simulink model "ALL_JP360_DBW_V6_5_1103"  (R2022a)
settings: Solver=FixedStepAuto  StartTime=0.0  StopTime=inf  FixedStep=0.01  RelTol=1e-3  EnableMultiTasking=on
model workspace (MAT data in the model file):
  g = 9.8
undefined symbols (not defined in the file or in its folder): canChannel, delta_v_p, IPM_Line_C0, IPM_Line_C1, IPM_Line_C2, IPM_Line_C3, M, M_p, MRR_ObjDistX, MRR_ObjDistY, MRR_ObjFusionCamID, MRR_ObjFusionSig, MRR_ObjID, MRR_ObjRelVelX, MRR_ObjRelVelY, MRR_ObjType, MRR_ObjUpdFlg, none, obj_vaild, untracktime, V, videoinput
libraries: canfdmsglib x230, canfdlib x76, slpidlib x24, simulink x18, dspstat3 x14, ctrlSharedLib x1, simulink_extras x1, imaqlib x1, realtime_pacer_lib x1, dspvision x1, visionsinks x1
(part 5 of 55)

== system ALL_JP360_DBW_V6_5_1103/MsgFromCAN/CCAN_GW_MsgFromCAN ==
  CCAN_GW_ABS_Sts_0x221FromInData : Inport  OutDataTypeStr=Bus:CAN_FD_MESSAGE_BUS
  CCAN_GW_ABS_Vspeed_0x601FromInData : Inport  Port=2  OutDataTypeStr=Bus:CAN_FD_MESSAGE_BUS
  CCAN_GW_ABS_WhlSpd_0x211FromInData : Inport  Port=3  OutDataTypeStr=Bus:CAN_FD_MESSAGE_BUS
  CCAN_GW_ADCU_0x538FromInData : Inport  Port=4  OutDataTypeStr=Bus:CAN_FD_MESSAGE_BUS
  CCAN_GW_ADCU_CanTSyn_0x570FromInData : Inport  Port=5  OutDataTypeStr=Bus:CAN_FD_MESSAGE_BUS
  CCAN_GW_BSD_0x275FromInData : Inport  Port=6  OutDataTypeStr=Bus:CAN_FD_MESSAGE_BUS
  CCAN_GW_EPS_0x260FromInData : Inport  Port=7  OutDataTypeStr=Bus:CAN_FD_MESSAGE_BUS
  CCAN_GW_EPS_Advanced_0x176FromInData : Inport  Port=8  OutDataTypeStr=Bus:CAN_FD_MESSAGE_BUS
  CCAN_GW_EPS_NM_0x5C2FromInData : Inport  Port=9  OutDataTypeStr=Bus:CAN_FD_MESSAGE_BUS
  CCAN_GW_ESP_Advanced_0x234FromInData : Inport  Port=10  OutDataTypeStr=Bus:CAN_FD_MESSAGE_BUS
  CCAN_GW_ESP_AxAy_0x242FromInData : Inport  Port=11  OutDataTypeStr=Bus:CAN_FD_MESSAGE_BUS
  CCAN_GW_ESP_Direction_0x235FromInData : Inport  Port=12  OutDataTypeStr=Bus:CAN_FD_MESSAGE_BUS
  CCAN_GW_ESP_OBD_Diag_0x600FromInData : Inport  Port=13  OutDataTypeStr=Bus:CAN_FD_MESSAGE_BUS
  CCAN_GW_ESP_Pressure_0x241FromInData : Inport  Port=14  OutDataTypeStr=Bus:CAN_FD_MESSAGE_BUS
  CCAN_GW_ESP_RAW_0x212FromInData : Inport  Port=15  OutDataTypeStr=Bus:CAN_FD_MESSAGE_BUS
  CCAN_GW_ESP_RPMF_0x213FromInData : Inport  Port=16  OutDataTypeStr=Bus:CAN_FD_MESSAGE_BUS
  CCAN_GW_ESP_RPMR_0x214FromInData : Inport  Port=17  OutDataTypeStr=Bus:CAN_FD_MESSAGE_BUS
  CCAN_GW_ESP_Status_0x243FromInData : Inport  Port=18  OutDataTypeStr=Bus:CAN_FD_MESSAGE_BUS
  CCAN_GW_ESP_Tq_0x217FromInData : Inport  Port=19  OutDataTypeStr=Bus:CAN_FD_MESSAGE_BUS
  CCAN_GW_GW_ESP_CCO_0x252FromInData : Inport  Port=20  OutDataTypeStr=Bus:CAN_FD_MESSAGE_BUS
  CCAN_GW_IPM_0x245FromInData : Inport  Port=21  OutDataTypeStr=Bus:CAN_FD_MESSAGE_BUS
  CCAN_GW_IPM_0x247FromInData : Inport  Port=22  OutDataTypeStr=Bus:CAN_FD_MESSAGE_BUS
  CCAN_GW_IPM_LeftLine_0x278FromInData : Inport  Port=23  OutDataTypeStr=Bus:CAN_FD_MESSAGE_BUS
  CCAN_GW_IPM_LeftLine_0x280FromInData : Inport  Port=24  OutDataTypeStr=Bus:CAN_FD_MESSAGE_BUS
  CCAN_GW_IPM_RightLine_0x490FromInData : Inport  Port=25  OutDataTypeStr=Bus:CAN_FD_MESSAGE_BUS
  CCAN_GW_IPM_RightLine_0x491FromInData : Inport  Port=26  OutDataTypeStr=Bus:CAN_FD_MESSAGE_BUS
  CCAN_GW_IPM_VLC_0x293FromInData : Inport  Port=27  OutDataTypeStr=Bus:CAN_FD_MESSAGE_BUS
  CCAN_GW_MRR_0x238FromInData : Inport  Port=28  OutDataTypeStr=Bus:CAN_FD_MESSAGE_BUS
  CCAN_GW_MRR_0x239FromInData : Inport  Port=29  OutDataTypeStr=Bus:CAN_FD_MESSAGE_BUS
  CCAN_GW_MRR_0x246FromInData : Inport  Port=30  OutDataTypeStr=Bus:CAN_FD_MESSAGE_BUS
  CCAN_GW_MRR_FRObj_0x279FromInData : Inport  Port=31  OutDataTypeStr=Bus:CAN_FD_MESSAGE_BUS
  CCAN_GW_MRR_LRObj_0x480FromInData : Inport  Port=32  OutDataTypeStr=Bus:CAN_FD_MESSAGE_BUS
  CCAN_GW_SAS_Sensor_0x175FromInData : Inport  Port=33  OutDataTypeStr=Bus:CAN_FD_MESSAGE_BUS
  CCAN_GW_SRR_FL_0x27BFromInData : Inport  Port=34  OutDataTypeStr=Bus:CAN_FD_MESSAGE_BUS
  CCAN_GW_SRR_RL_0x27AFromInData : Inport  Port=35  OutDataTypeStr=Bus:CAN_FD_MESSAGE_BUS
  CCAN_GW_ABS_Sts_0x221 : Subsystem  Commented=on  TreatAsAtomicUnit=on
  CCAN_GW_ABS_Vspeed_0x601 : Subsystem  Commented=on  TreatAsAtomicUnit=on
  CCAN_GW_ABS_WhlSpd_0x211 : Subsystem  Commented=on  TreatAsAtomicUnit=on
  CCAN_GW_ADCU_0x538 : Subsystem  Commented=on  TreatAsAtomicUnit=on
  CCAN_GW_ADCU_CanTSyn_0x570 : Subsystem  Commented=on  TreatAsAtomicUnit=on
  CCAN_GW_BSD_0x275 : Subsystem  Commented=on  TreatAsAtomicUnit=on
  CCAN_GW_EPS_0x260 : Subsystem  Commented=on  TreatAsAtomicUnit=on
  CCAN_GW_EPS_Advanced_0x176 : Subsystem  Commented=on  TreatAsAtomicUnit=on
  CCAN_GW_EPS_NM_0x5C2 : Subsystem  Commented=on  TreatAsAtomicUnit=on
  CCAN_GW_ESP_Advanced_0x234 : Subsystem  Commented=on  TreatAsAtomicUnit=on
  CCAN_GW_ESP_AxAy_0x242 : Subsystem  Commented=on  TreatAsAtomicUnit=on
  CCAN_GW_ESP_Direction_0x235 : Subsystem  Commented=on  TreatAsAtomicUnit=on
  CCAN_GW_ESP_OBD_Diag_0x600 : Subsystem  Commented=on  TreatAsAtomicUnit=on
  CCAN_GW_ESP_Pressure_0x241 : Subsystem  Commented=on  TreatAsAtomicUnit=on
  CCAN_GW_ESP_RAW_0x212 : Subsystem  Commented=on  TreatAsAtomicUnit=on
  CCAN_GW_ESP_RPMF_0x213 : Subsystem  Commented=on  TreatAsAtomicUnit=on
  CCAN_GW_ESP_RPMR_0x214 : Subsystem  Commented=on  TreatAsAtomicUnit=on
  CCAN_GW_ESP_Status_0x243 : Subsystem  Commented=on  TreatAsAtomicUnit=on
  CCAN_GW_ESP_Tq_0x217 : Subsystem  Commented=on  TreatAsAtomicUnit=on
  CCAN_GW_GW_ESP_CCO_0x252 : Subsystem  Commented=on  TreatAsAtomicUnit=on
  CCAN_GW_IPM_0x245 : Subsystem  Commented=on  TreatAsAtomicUnit=on
  CCAN_GW_IPM_0x247 : Subsystem  Commented=on  TreatAsAtomicUnit=on
  CCAN_GW_IPM_LeftLine_0x278 : Subsystem  Commented=on  TreatAsAtomicUnit=on
  CCAN_GW_IPM_LeftLine_0x280 : Subsystem  Commented=on  TreatAsAtomicUnit=on
  CCAN_GW_IPM_RightLine_0x490 : Subsystem  Commented=on  TreatAsAtomicUnit=on
  CCAN_GW_IPM_RightLine_0x491 : Subsystem  Commented=on  TreatAsAtomicUnit=on
  CCAN_GW_IPM_VLC_0x293 : Subsystem  Commented=on  TreatAsAtomicUnit=on
  CCAN_GW_MRR_0x238 : Subsystem  Commented=on  TreatAsAtomicUnit=on
  CCAN_GW_MRR_0x239 : Subsystem  Commented=on  TreatAsAtomicUnit=on
  CCAN_GW_MRR_0x246 : Subsystem  TreatAsAtomicUnit=on
  CCAN_GW_MRR_FRObj_0x279 : Subsystem  TreatAsAtomicUnit=on
  CCAN_GW_MRR_LRObj_0x480 : Subsystem  Commented=on  TreatAsAtomicUnit=on
  CCAN_GW_SAS_Sensor_0x175 : Subsystem  Commented=on  TreatAsAtomicUnit=on
  CCAN_GW_SRR_FL_0x27B : Subsystem  Commented=on  TreatAsAtomicUnit=on
  CCAN_GW_SRR_RL_0x27A : Subsystem  Commented=on  TreatAsAtomicUnit=on
  CCAN_GW_ABS_Sts_0x221FromOutData : Outport  OutDataTypeStr=Bus:CCAN_GW_ABS_Sts_0x221
  CCAN_GW_ABS_Vspeed_0x601FromOutData : Outport  Port=2  OutDataTypeStr=Bus:CCAN_GW_ABS_Vspeed_0x601
  CCAN_GW_ABS_WhlSpd_0x211FromOutData : Outport  Port=3  OutDataTypeStr=Bus:CCAN_GW_ABS_WhlSpd_0x211
  CCAN_GW_ADCU_0x538FromOutData : Outport  Port=4  OutDataTypeStr=Bus:CCAN_GW_ADCU_0x538
  CCAN_GW_ADCU_CanTSyn_0x570FromOutData : Outport  Port=5  OutDataTypeStr=Bus:CCAN_GW_ADCU_CanTSyn_0x570
  CCAN_GW_BSD_0x275FromOutData : Outport  Port=6  OutDataTypeStr=Bus:CCAN_GW_BSD_0x275
  CCAN_GW_EPS_0x260FromOutData : Outport  Port=7  OutDataTypeStr=Bus:CCAN_GW_EPS_0x260
  CCAN_GW_EPS_Advanced_0x176FromOutData : Outport  Port=8  OutDataTypeStr=Bus:CCAN_GW_EPS_Advanced_0x176
  CCAN_GW_EPS_NM_0x5C2FromOutData : Outport  Port=9  OutDataTypeStr=Bus:CCAN_GW_EPS_NM_0x5C2
  CCAN_GW_ESP_Advanced_0x234FromOutData : Outport  Port=10  OutDataTypeStr=Bus:CCAN_GW_ESP_Advanced_0x234
  CCAN_GW_ESP_AxAy_0x242FromOutData : Outport  Port=11  OutDataTypeStr=Bus:CCAN_GW_ESP_AxAy_0x242
  CCAN_GW_ESP_Direction_0x235FromOutData : Outport  Port=12  OutDataTypeStr=Bus:CCAN_GW_ESP_Direction_0x235
  CCAN_GW_ESP_OBD_Diag_0x600FromOutData : Outport  Port=13  OutDataTypeStr=Bus:CCAN_GW_ESP_OBD_Diag_0x600
  CCAN_GW_ESP_Pressure_0x241FromOutData : Outport  Port=14  OutDataTypeStr=Bus:CCAN_GW_ESP_Pressure_0x241
  CCAN_GW_ESP_RAW_0x212FromOutData : Outport  Port=15  OutDataTypeStr=Bus:CCAN_GW_ESP_RAW_0x212
  CCAN_GW_ESP_RPMF_0x213FromOutData : Outport  Port=16  OutDataTypeStr=Bus:CCAN_GW_ESP_RPMF_0x213
  CCAN_GW_ESP_RPMR_0x214FromOutData : Outport  Port=17  OutDataTypeStr=Bus:CCAN_GW_ESP_RPMR_0x214
  CCAN_GW_ESP_Status_0x243FromOutData : Outport  Port=18  OutDataTypeStr=Bus:CCAN_GW_ESP_Status_0x243
  CCAN_GW_ESP_Tq_0x217FromOutData : Outport  Port=19  OutDataTypeStr=Bus:CCAN_GW_ESP_Tq_0x217
  CCAN_GW_GW_ESP_CCO_0x252FromOutData : Outport  Port=20  OutDataTypeStr=Bus:CCAN_GW_GW_ESP_CCO_0x252
  CCAN_GW_IPM_0x245FromOutData : Outport  Port=21  OutDataTypeStr=Bus:CCAN_GW_IPM_0x245
  CCAN_GW_IPM_0x247FromOutData : Outport  Port=22  OutDataTypeStr=Bus:CCAN_GW_IPM_0x247
  CCAN_GW_IPM_LeftLine_0x278FromOutData : Outport  Port=23  OutDataTypeStr=Bus:CCAN_GW_IPM_LeftLine_0x278
  CCAN_GW_IPM_LeftLine_0x280FromOutData : Outport  Port=24  OutDataTypeStr=Bus:CCAN_GW_IPM_LeftLine_0x280
  CCAN_GW_IPM_RightLine_0x490FromOutData : Outport  Port=25  OutDataTypeStr=Bus:CCAN_GW_IPM_RightLine_0x490
  CCAN_GW_IPM_RightLine_0x491FromOutData : Outport  Port=26  OutDataTypeStr=Bus:CCAN_GW_IPM_RightLine_0x491
  CCAN_GW_IPM_VLC_0x293FromOutData : Outport  Port=27  OutDataTypeStr=Bus:CCAN_GW_IPM_VLC_0x293
  CCAN_GW_MRR_0x238FromOutData : Outport  Port=28  OutDataTypeStr=Bus:CCAN_GW_MRR_0x238
  CCAN_GW_MRR_0x239FromOutData : Outport  Port=29  OutDataTypeStr=Bus:CCAN_GW_MRR_0x239
  CCAN_GW_MRR_0x246FromOutData : Outport  Port=30  OutDataTypeStr=Bus:CCAN_GW_MRR_0x246
  CCAN_GW_MRR_FRObj_0x279FromOutData : Outport  Port=31  OutDataTypeStr=Bus:CCAN_GW_MRR_FRObj_0x279
  CCAN_GW_MRR_LRObj_0x480FromOutData : Outport  Port=32  OutDataTypeStr=Bus:CCAN_GW_MRR_LRObj_0x480
  CCAN_GW_SAS_Sensor_0x175FromOutData : Outport  Port=33  OutDataTypeStr=Bus:CCAN_GW_SAS_Sensor_0x175
  CCAN_GW_SRR_FL_0x27BFromOutData : Outport  Port=34  OutDataTypeStr=Bus:CCAN_GW_SRR_FL_0x27B
  CCAN_GW_SRR_RL_0x27AFromOutData : Outport  Port=35  OutDataTypeStr=Bus:CCAN_GW_SRR_RL_0x27A
  wires:
  CCAN_GW_ABS_Sts_0x221/1(CCAN_GW_ABS_Sts_0x221FromOutData) -> CCAN_GW_ABS_Sts_0x221FromOutData/1  "CCAN_GW_ABS_Sts_0x221FromOutData"
  CCAN_GW_ABS_Sts_0x221FromInData/1 -> CCAN_GW_ABS_Sts_0x221/1(CCAN_GW_ABS_Sts_0x221FromInData)  "CCAN_GW_ABS_Sts_0x221FromInData"
  CCAN_GW_ABS_Vspeed_0x601/1(CCAN_GW_ABS_Vspeed_0x601FromOutData) -> CCAN_GW_ABS_Vspeed_0x601FromOutData/1  "CCAN_GW_ABS_Vspeed_0x601FromOutData"
  CCAN_GW_ABS_Vspeed_0x601FromInData/1 -> CCAN_GW_ABS_Vspeed_0x601/1(CCAN_GW_ABS_Vspeed_0x601FromInData)  "CCAN_GW_ABS_Vspeed_0x601FromInData"
  CCAN_GW_ABS_WhlSpd_0x211/1(CCAN_GW_ABS_WhlSpd_0x211FromOutData) -> CCAN_GW_ABS_WhlSpd_0x211FromOutData/1  "CCAN_GW_ABS_WhlSpd_0x211FromOutData"
  CCAN_GW_ABS_WhlSpd_0x211FromInData/1 -> CCAN_GW_ABS_WhlSpd_0x211/1(CCAN_GW_ABS_WhlSpd_0x211FromInData)  "CCAN_GW_ABS_WhlSpd_0x211FromInData"
  CCAN_GW_ADCU_0x538/1(CCAN_GW_ADCU_0x538FromOutData) -> CCAN_GW_ADCU_0x538FromOutData/1  "CCAN_GW_ADCU_0x538FromOutData"
  CCAN_GW_ADCU_0x538FromInData/1 -> CCAN_GW_ADCU_0x538/1(CCAN_GW_ADCU_0x538FromInData)  "CCAN_GW_ADCU_0x538FromInData"
  CCAN_GW_ADCU_CanTSyn_0x570/1(CCAN_GW_ADCU_CanTSyn_0x570FromOutData) -> CCAN_GW_ADCU_CanTSyn_0x570FromOutData/1  "CCAN_GW_ADCU_CanTSyn_0x570FromOutData"
  CCAN_GW_ADCU_CanTSyn_0x570FromInData/1 -> CCAN_GW_ADCU_CanTSyn_0x570/1(CCAN_GW_ADCU_CanTSyn_0x570FromInData)  "CCAN_GW_ADCU_CanTSyn_0x570FromInData"
  CCAN_GW_BSD_0x275/1(CCAN_GW_BSD_0x275FromOutData) -> CCAN_GW_BSD_0x275FromOutData/1  "CCAN_GW_BSD_0x275FromOutData"
  CCAN_GW_BSD_0x275FromInData/1 -> CCAN_GW_BSD_0x275/1(CCAN_GW_BSD_0x275FromInData)  "CCAN_GW_BSD_0x275FromInData"
  CCAN_GW_EPS_0x260/1(CCAN_GW_EPS_0x260FromOutData) -> CCAN_GW_EPS_0x260FromOutData/1  "CCAN_GW_EPS_0x260FromOutData"
  CCAN_GW_EPS_0x260FromInData/1 -> CCAN_GW_EPS_0x260/1(CCAN_GW_EPS_0x260FromInData)  "CCAN_GW_EPS_0x260FromInData"
  CCAN_GW_EPS_Advanced_0x176/1(CCAN_GW_EPS_Advanced_0x176FromOutData) -> CCAN_GW_EPS_Advanced_0x176FromOutData/1  "CCAN_GW_EPS_Advanced_0x176FromOutData"
  CCAN_GW_EPS_Advanced_0x176FromInData/1 -> CCAN_GW_EPS_Advanced_0x176/1(CCAN_GW_EPS_Advanced_0x176FromInData)  "CCAN_GW_EPS_Advanced_0x176FromInData"
  CCAN_GW_EPS_NM_0x5C2/1(CCAN_GW_EPS_NM_0x5C2FromOutData) -> CCAN_GW_EPS_NM_0x5C2FromOutData/1  "CCAN_GW_EPS_NM_0x5C2FromOutData"
  CCAN_GW_EPS_NM_0x5C2FromInData/1 -> CCAN_GW_EPS_NM_0x5C2/1(CCAN_GW_EPS_NM_0x5C2FromInData)  "CCAN_GW_EPS_NM_0x5C2FromInData"
  CCAN_GW_ESP_Advanced_0x234/1(CCAN_GW_ESP_Advanced_0x234FromOutData) -> CCAN_GW_ESP_Advanced_0x234FromOutData/1  "CCAN_GW_ESP_Advanced_0x234FromOutData"
  CCAN_GW_ESP_Advanced_0x234FromInData/1 -> CCAN_GW_ESP_Advanced_0x234/1(CCAN_GW_ESP_Advanced_0x234FromInData)  "CCAN_GW_ESP_Advanced_0x234FromInData"
  CCAN_GW_ESP_AxAy_0x242/1(CCAN_GW_ESP_AxAy_0x242FromOutData) -> CCAN_GW_ESP_AxAy_0x242FromOutData/1  "CCAN_GW_ESP_AxAy_0x242FromOutData"
  CCAN_GW_ESP_AxAy_0x242FromInData/1 -> CCAN_GW_ESP_AxAy_0x242/1(CCAN_GW_ESP_AxAy_0x242FromInData)  "CCAN_GW_ESP_AxAy_0x242FromInData"
  CCAN_GW_ESP_Direction_0x235/1(CCAN_GW_ESP_Direction_0x235FromOutData) -> CCAN_GW_ESP_Direction_0x235FromOutData/1  "CCAN_GW_ESP_Direction_0x235FromOutData"
  CCAN_GW_ESP_Direction_0x235FromInData/1 -> CCAN_GW_ESP_Direction_0x235/1(CCAN_GW_ESP_Direction_0x235FromInData)  "CCAN_GW_ESP_Direction_0x235FromInData"
  CCAN_GW_ESP_OBD_Diag_0x600/1(CCAN_GW_ESP_OBD_Diag_0x600FromOutData) -> CCAN_GW_ESP_OBD_Diag_0x600FromOutData/1  "CCAN_GW_ESP_OBD_Diag_0x600FromOutData"
  CCAN_GW_ESP_OBD_Diag_0x600FromInData/1 -> CCAN_GW_ESP_OBD_Diag_0x600/1(CCAN_GW_ESP_OBD_Diag_0x600FromInData)  "CCAN_GW_ESP_OBD_Diag_0x600FromInData"
  CCAN_GW_ESP_Pressure_0x241/1(CCAN_GW_ESP_Pressure_0x241FromOutData) -> CCAN_GW_ESP_Pressure_0x241FromOutData/1  "CCAN_GW_ESP_Pressure_0x241FromOutData"
  CCAN_GW_ESP_Pressure_0x241FromInData/1 -> CCAN_GW_ESP_Pressure_0x241/1(CCAN_GW_ESP_Pressure_0x241FromInData)  "CCAN_GW_ESP_Pressure_0x241FromInData"
  CCAN_GW_ESP_RAW_0x212/1(CCAN_GW_ESP_RAW_0x212FromOutData) -> CCAN_GW_ESP_RAW_0x212FromOutData/1  "CCAN_GW_ESP_RAW_0x212FromOutData"
  CCAN_GW_ESP_RAW_0x212FromInData/1 -> CCAN_GW_ESP_RAW_0x212/1(CCAN_GW_ESP_RAW_0x212FromInData)  "CCAN_GW_ESP_RAW_0x212FromInData"
  CCAN_GW_ESP_RPMF_0x213/1(CCAN_GW_ESP_RPMF_0x213FromOutData) -> CCAN_GW_ESP_RPMF_0x213FromOutData/1  "CCAN_GW_ESP_RPMF_0x213FromOutData"
  CCAN_GW_ESP_RPMF_0x213FromInData/1 -> CCAN_GW_ESP_RPMF_0x213/1(CCAN_GW_ESP_RPMF_0x213FromInData)  "CCAN_GW_ESP_RPMF_0x213FromInData"
  CCAN_GW_ESP_RPMR_0x214/1(CCAN_GW_ESP_RPMR_0x214FromOutData) -> CCAN_GW_ESP_RPMR_0x214FromOutData/1  "CCAN_GW_ESP_RPMR_0x214FromOutData"
  CCAN_GW_ESP_RPMR_0x214FromInData/1 -> CCAN_GW_ESP_RPMR_0x214/1(CCAN_GW_ESP_RPMR_0x214FromInData)  "CCAN_GW_ESP_RPMR_0x214FromInData"
  CCAN_GW_ESP_Status_0x243/1(CCAN_GW_ESP_Status_0x243FromOutData) -> CCAN_GW_ESP_Status_0x243FromOutData/1  "CCAN_GW_ESP_Status_0x243FromOutData"
  CCAN_GW_ESP_Status_0x243FromInData/1 -> CCAN_GW_ESP_Status_0x243/1(CCAN_GW_ESP_Status_0x243FromInData)  "CCAN_GW_ESP_Status_0x243FromInData"
  CCAN_GW_ESP_Tq_0x217/1(CCAN_GW_ESP_Tq_0x217FromOutData) -> CCAN_GW_ESP_Tq_0x217FromOutData/1  "CCAN_GW_ESP_Tq_0x217FromOutData"
  CCAN_GW_ESP_Tq_0x217FromInData/1 -> CCAN_GW_ESP_Tq_0x217/1(CCAN_GW_ESP_Tq_0x217FromInData)  "CCAN_GW_ESP_Tq_0x217FromInData"
  CCAN_GW_GW_ESP_CCO_0x252/1(CCAN_GW_GW_ESP_CCO_0x252FromOutData) -> CCAN_GW_GW_ESP_CCO_0x252FromOutData/1  "CCAN_GW_GW_ESP_CCO_0x252FromOutData"
  CCAN_GW_GW_ESP_CCO_0x252FromInData/1 -> CCAN_GW_GW_ESP_CCO_0x252/1(CCAN_GW_GW_ESP_CCO_0x252FromInData)  "CCAN_GW_GW_ESP_CCO_0x252FromInData"
  CCAN_GW_IPM_0x245/1(CCAN_GW_IPM_0x245FromOutData) -> CCAN_GW_IPM_0x245FromOutData/1  "CCAN_GW_IPM_0x245FromOutData"
  CCAN_GW_IPM_0x245FromInData/1 -> CCAN_GW_IPM_0x245/1(CCAN_GW_IPM_0x245FromInData)  "CCAN_GW_IPM_0x245FromInData"
  CCAN_GW_IPM_0x247/1(CCAN_GW_IPM_0x247FromOutData) -> CCAN_GW_IPM_0x247FromOutData/1  "CCAN_GW_IPM_0x247FromOutData"
  CCAN_GW_IPM_0x247FromInData/1 -> CCAN_GW_IPM_0x247/1(CCAN_GW_IPM_0x247FromInData)  "CCAN_GW_IPM_0x247FromInData"
  CCAN_GW_IPM_LeftLine_0x278/1(CCAN_GW_IPM_LeftLine_0x278FromOutData) -> CCAN_GW_IPM_LeftLine_0x278FromOutData/1  "CCAN_GW_IPM_LeftLine_0x278FromOutData"
  CCAN_GW_IPM_LeftLine_0x278FromInData/1 -> CCAN_GW_IPM_LeftLine_0x278/1(CCAN_GW_IPM_LeftLine_0x278FromInData)  "CCAN_GW_IPM_LeftLine_0x278FromInData"
  CCAN_GW_IPM_LeftLine_0x280/1(CCAN_GW_IPM_LeftLine_0x280FromOutData) -> CCAN_GW_IPM_LeftLine_0x280FromOutData/1  "CCAN_GW_IPM_LeftLine_0x280FromOutData"
  CCAN_GW_IPM_LeftLine_0x280FromInData/1 -> CCAN_GW_IPM_LeftLine_0x280/1(CCAN_GW_IPM_LeftLine_0x280FromInData)  "CCAN_GW_IPM_LeftLine_0x280FromInData"
  CCAN_GW_IPM_RightLine_0x490/1(CCAN_GW_IPM_RightLine_0x490FromOutData) -> CCAN_GW_IPM_RightLine_0x490FromOutData/1  "CCAN_GW_IPM_RightLine_0x490FromOutData"
  CCAN_GW_IPM_RightLine_0x490FromInData/1 -> CCAN_GW_IPM_RightLine_0x490/1(CCAN_GW_IPM_RightLine_0x490FromInData)  "CCAN_GW_IPM_RightLine_0x490FromInData"
  CCAN_GW_IPM_RightLine_0x491/1(CCAN_GW_IPM_RightLine_0x491FromOutData) -> CCAN_GW_IPM_RightLine_0x491FromOutData/1  "CCAN_GW_IPM_RightLine_0x491FromOutData"
  CCAN_GW_IPM_RightLine_0x491FromInData/1 -> CCAN_GW_IPM_RightLine_0x491/1(CCAN_GW_IPM_RightLine_0x491FromInData)  "CCAN_GW_IPM_RightLine_0x491FromInData"
  CCAN_GW_IPM_VLC_0x293/1(CCAN_GW_IPM_VLC_0x293FromOutData) -> CCAN_GW_IPM_VLC_0x293FromOutData/1  "CCAN_GW_IPM_VLC_0x293FromOutData"
  CCAN_GW_IPM_VLC_0x293FromInData/1 -> CCAN_GW_IPM_VLC_0x293/1(CCAN_GW_IPM_VLC_0x293FromInData)  "CCAN_GW_IPM_VLC_0x293FromInData"
  CCAN_GW_MRR_0x238/1(CCAN_GW_MRR_0x238FromOutData) -> CCAN_GW_MRR_0x238FromOutData/1  "CCAN_GW_MRR_0x238FromOutData"
  CCAN_GW_MRR_0x238FromInData/1 -> CCAN_GW_MRR_0x238/1(CCAN_GW_MRR_0x238FromInData)  "CCAN_GW_MRR_0x238FromInData"
  CCAN_GW_MRR_0x239/1(CCAN_GW_MRR_0x239FromOutData) -> CCAN_GW_MRR_0x239FromOutData/1  "CCAN_GW_MRR_0x239FromOutData"
  CCAN_GW_MRR_0x239FromInData/1 -> CCAN_GW_MRR_0x239/1(CCAN_GW_MRR_0x239FromInData)  "CCAN_GW_MRR_0x239FromInData"
  CCAN_GW_MRR_0x246/1(CCAN_GW_MRR_0x246FromOutData) -> CCAN_GW_MRR_0x246FromOutData/1  "CCAN_GW_MRR_0x246FromOutData"
  CCAN_GW_MRR_0x246FromInData/1 -> CCAN_GW_MRR_0x246/1(CCAN_GW_MRR_0x246FromInData)  "CCAN_GW_MRR_0x246FromInData"
  CCAN_GW_MRR_FRObj_0x279/1(CCAN_GW_MRR_FRObj_0x279FromOutData) -> CCAN_GW_MRR_FRObj_0x279FromOutData/1  "CCAN_GW_MRR_FRObj_0x279FromOutData"
  CCAN_GW_MRR_FRObj_0x279FromInData/1 -> CCAN_GW_MRR_FRObj_0x279/1(CCAN_GW_MRR_FRObj_0x279FromInData)  "CCAN_GW_MRR_FRObj_0x279FromInData"
  CCAN_GW_MRR_LRObj_0x480/1(CCAN_GW_MRR_LRObj_0x480FromOutData) -> CCAN_GW_MRR_LRObj_0x480FromOutData/1  "CCAN_GW_MRR_LRObj_0x480FromOutData"
  CCAN_GW_MRR_LRObj_0x480FromInData/1 -> CCAN_GW_MRR_LRObj_0x480/1(CCAN_GW_MRR_LRObj_0x480FromInData)  "CCAN_GW_MRR_LRObj_0x480FromInData"
  CCAN_GW_SAS_Sensor_0x175/1(CCAN_GW_SAS_Sensor_0x175FromOutData) -> CCAN_GW_SAS_Sensor_0x175FromOutData/1  "CCAN_GW_SAS_Sensor_0x175FromOutData"
  CCAN_GW_SAS_Sensor_0x175FromInData/1 -> CCAN_GW_SAS_Sensor_0x175/1(CCAN_GW_SAS_Sensor_0x175FromInData)  "CCAN_GW_SAS_Sensor_0x175FromInData"
  CCAN_GW_SRR_FL_0x27B/1(CCAN_GW_SRR_FL_0x27BFromOutData) -> CCAN_GW_SRR_FL_0x27BFromOutData/1  "CCAN_GW_SRR_FL_0x27BFromOutData"
  CCAN_GW_SRR_FL_0x27BFromInData/1 -> CCAN_GW_SRR_FL_0x27B/1(CCAN_GW_SRR_FL_0x27BFromInData)  "CCAN_GW_SRR_FL_0x27BFromInData"
  CCAN_GW_SRR_RL_0x27A/1(CCAN_GW_SRR_RL_0x27AFromOutData) -> CCAN_GW_SRR_RL_0x27AFromOutData/1  "CCAN_GW_SRR_RL_0x27AFromOutData"
  CCAN_GW_SRR_RL_0x27AFromInData/1 -> CCAN_GW_SRR_RL_0x27A/1(CCAN_GW_SRR_RL_0x27AFromInData)  "CCAN_GW_SRR_RL_0x27AFromInData"

== system ALL_JP360_DBW_V6_5_1103/MsgFromCAN/IPM_Line_data ==
  CAN FD Receive1 : canfdlib/CAN FD Receive  BlockHandle=84597.0006  Device=Vector VN1640A 1 (Channel 4)  ObjConstructor=canChannel('Vector', 'VN1640A 1', 4, 'ProtocolMode', 'CAN FD')  EnableStandardIDsFilter=off  StdIDsCombo=Allow only  StandardIDs=1600  EnableExtendedIDsFilter=off  ExtIDsCombo=Allow all  ExtendedIDs=0  SampleTime=0.01  MsgsPerTimestep=all  InternalFilterUpdateStatus=on  BusOutput=on
      settings: SourceProductBaseCode=VN
  CAN FD Receive2 : canfdlib/CAN FD Receive  BlockHandle=84600.0006  Device=Vector VN1640A 1 (Channel 4)  ObjConstructor=canChannel('Vector', 'VN1640A 1', 4, 'ProtocolMode', 'CAN FD')  EnableStandardIDsFilter=off  StdIDsCombo=Allow only  StandardIDs=1601  EnableExtendedIDsFilter=off  ExtIDsCombo=Allow all  ExtendedIDs=0  SampleTime=0.01  MsgsPerTimestep=all  InternalFilterUpdateStatus=on  BusOutput=on
      settings: SourceProductBaseCode=VN
  CAN FD Receive3 : canfdlib/CAN FD Receive  BlockHandle=84603.0006  Device=Vector VN1640A 1 (Channel 4)  ObjConstructor=canChannel('Vector', 'VN1640A 1', 4, 'ProtocolMode', 'CAN FD')  EnableStandardIDsFilter=off  StdIDsCombo=Allow only  StandardIDs=1602  EnableExtendedIDsFilter=off  ExtIDsCombo=Allow all  ExtendedIDs=0  SampleTime=0.01  MsgsPerTimestep=all  InternalFilterUpdateStatus=on  BusOutput=on
      settings: SourceProductBaseCode=VN
  CAN FD Receive4 : canfdlib/CAN FD Receive  BlockHandle=84606.0006  Device=Vector VN1640A 1 (Channel 4)  ObjConstructor=canChannel('Vector', 'VN1640A 1', 4, 'ProtocolMode', 'CAN FD')  EnableStandardIDsFilter=off  StdIDsCombo=Allow only  StandardIDs=1603  EnableExtendedIDsFilter=off  ExtIDsCombo=Allow all  ExtendedIDs=0  SampleTime=0.01  MsgsPerTimestep=all  InternalFilterUpdateStatus=on  BusOutput=on
      settings: SourceProductBaseCode=VN
  Terminator{16..19} (4 alike) : Terminator
  VR_ADCU_IPM_Line_01_0x640FromInData : Outport
  VR_ADCU_IPM_Line_02_0x641FromInData : Outport  Port=2
  VR_ADCU_IPM_Line_03_0x642FromInData : Outport  Port=3
  VR_ADCU_IPM_Line_04_0x643FromInData : Outport  Port=4
  wires:
  CAN FD Receive4/1 -> Terminator19/1
  CAN FD Receive3/1 -> Terminator18/1
  CAN FD Receive3/2 -> VR_ADCU_IPM_Line_03_0x642FromInData/1
  CAN FD Receive1/1 -> Terminator16/1
  CAN FD Receive4/2 -> VR_ADCU_IPM_Line_04_0x643FromInData/1
  CAN FD Receive2/1 -> Terminator17/1
  CAN FD Receive2/2 -> VR_ADCU_IPM_Line_02_0x641FromInData/1
  CAN FD Receive1/2 -> VR_ADCU_IPM_Line_01_0x640FromInData/1

== system ALL_JP360_DBW_V6_5_1103/MsgFromCAN/IPM_Obj_data ==
  CAN FD Receive1 : canfdlib/CAN FD Receive  BlockHandle=84647.0004  Device=Vector VN1640A 1 (Channel 4)  ObjConstructor=canChannel('Vector', 'VN1640A 1', 4, 'ProtocolMode', 'CAN FD')  EnableStandardIDsFilter=off  StdIDsCombo=Allow only  StandardIDs=1616  EnableExtendedIDsFilter=off  ExtIDsCombo=Allow all  ExtendedIDs=0  SampleTime=0.01  MsgsPerTimestep=all  InternalFilterUpdateStatus=on  BusOutput=on
      settings: SourceProductBaseCode=VN
  CAN FD Receive10 : canfdlib/CAN FD Receive  BlockHandle=84650.0004  Device=Vector VN1640A 1 (Channel 4)  ObjConstructor=canChannel('Vector', 'VN1640A 1', 4, 'ProtocolMode', 'CAN FD')  EnableStandardIDsFilter=off  StdIDsCombo=Allow only  StandardIDs=1625  EnableExtendedIDsFilter=off  ExtIDsCombo=Allow all  ExtendedIDs=0  SampleTime=0.01  MsgsPerTimestep=all  InternalFilterUpdateStatus=on  BusOutput=on
      settings: SourceProductBaseCode=VN
  CAN FD Receive11 : canfdlib/CAN FD Receive  BlockHandle=84653.0004  Device=Vector VN1640A 1 (Channel 4)  ObjConstructor=canChannel('Vector', 'VN1640A 1', 4, 'ProtocolMode', 'CAN FD')  EnableStandardIDsFilter=off  StdIDsCombo=Allow only  StandardIDs=1626  EnableExtendedIDsFilter=off  ExtIDsCombo=Allow all  ExtendedIDs=0  SampleTime=0.01  MsgsPerTimestep=all  InternalFilterUpdateStatus=on  BusOutput=on
      settings: SourceProductBaseCode=VN
  CAN FD Receive12 : canfdlib/CAN FD Receive  BlockHandle=84656.0005  Device=Vector VN1640A 1 (Channel 4)  ObjConstructor=canChannel('Vector', 'VN1640A 1', 4, 'ProtocolMode', 'CAN FD')  EnableStandardIDsFilter=off  StdIDsCombo=Allow only  StandardIDs=1627  EnableExtendedIDsFilter=off  ExtIDsCombo=Allow all  ExtendedIDs=0  SampleTime=0.01  MsgsPerTimestep=all  InternalFilterUpdateStatus=on  BusOutput=on
      settings: SourceProductBaseCode=VN
  CAN FD Receive13 : canfdlib/CAN FD Receive  BlockHandle=84659.0012  Device=Vector VN1640A 1 (Channel 4)  ObjConstructor=canChannel('Vector', 'VN1640A 1', 4, 'ProtocolMode', 'CAN FD')  EnableStandardIDsFilter=off  StdIDsCombo=Allow only  StandardIDs=1628  EnableExtendedIDsFilter=off  ExtIDsCombo=Allow all  ExtendedIDs=0  SampleTime=0.01  MsgsPerTimestep=all  InternalFilterUpdateStatus=on  BusOutput=on
      settings: SourceProductBaseCode=VN
  CAN FD Receive14 : canfdlib/CAN FD Receive  BlockHandle=84662.0005  Device=Vector VN1640A 1 (Channel 4)  ObjConstructor=canChannel('Vector', 'VN1640A 1', 4, 'ProtocolMode', 'CAN FD')  EnableStandardIDsFilter=off  StdIDsCombo=Allow only  StandardIDs=1629  EnableExtendedIDsFilter=off  ExtIDsCombo=Allow all  ExtendedIDs=0  SampleTime=0.01  MsgsPerTimestep=all  InternalFilterUpdateStatus=on  BusOutput=on
      settings: SourceProductBaseCode=VN
  CAN FD Receive15 : canfdlib/CAN FD Receive  BlockHandle=84665.0004  Device=Vector VN1640A 1 (Channel 4)  ObjConstructor=canChannel('Vector', 'VN1640A 1', 4, 'ProtocolMode', 'CAN FD')  EnableStandardIDsFilter=off  StdIDsCombo=Allow only  StandardIDs=1630  EnableExtendedIDsFilter=off  ExtIDsCombo=Allow all  ExtendedIDs=0  SampleTime=0.01  MsgsPerTimestep=all  InternalFilterUpdateStatus=on  BusOutput=on
      settings: SourceProductBaseCode=VN
  CAN FD Receive16 : canfdlib/CAN FD Receive  BlockHandle=84668.0004  Device=Vector VN1640A 1 (Channel 4)  ObjConstructor=canChannel('Vector', 'VN1640A 1', 4, 'ProtocolMode', 'CAN FD')  EnableStandardIDsFilter=off  StdIDsCombo=Allow only  StandardIDs=1631  EnableExtendedIDsFilter=off  ExtIDsCombo=Allow all  ExtendedIDs=0  SampleTime=0.01  MsgsPerTimestep=all  InternalFilterUpdateStatus=on  BusOutput=on
      settings: SourceProductBaseCode=VN
  CAN FD Receive17 : canfdlib/CAN FD Receive  BlockHandle=84671.0004  Device=Vector VN1640A 1 (Channel 4)  ObjConstructor=canChannel('Vector', 'VN1640A 1', 4, 'ProtocolMode', 'CAN FD')  EnableStandardIDsFilter=off  StdIDsCombo=Allow only  StandardIDs=1632  EnableExtendedIDsFilter=off  ExtIDsCombo=Allow all  ExtendedIDs=0  SampleTime=0.01  MsgsPerTimestep=all  InternalFilterUpdateStatus=on  BusOutput=on
      settings: SourceProductBaseCode=VN
  CAN FD Receive18 : canfdlib/CAN FD Receive  BlockHandle=84674.0004  Device=Vector VN1640A 1 (Channel 4)  ObjConstructor=canChannel('Vector', 'VN1640A 1', 4, 'ProtocolMode', 'CAN FD')  EnableStandardIDsFilter=off  StdIDsCombo=Allow only  StandardIDs=1633  EnableExtendedIDsFilter=off  ExtIDsCombo=Allow all  ExtendedIDs=0  SampleTime=0.01  MsgsPerTimestep=all  InternalFilterUpdateStatus=on  BusOutput=on
      settings: SourceProductBaseCode=VN
  CAN FD Receive19 : canfdlib/CAN FD Receive  BlockHandle=84677.0004  Device=Vector VN1640A 1 (Channel 4)  ObjConstructor=canChannel('Vector', 'VN1640A 1', 4, 'ProtocolMode', 'CAN FD')  EnableStandardIDsFilter=off  StdIDsCombo=Allow only  StandardIDs=1634  EnableExtendedIDsFilter=off  ExtIDsCombo=Allow all  ExtendedIDs=0  SampleTime=0.01  MsgsPerTimestep=all  InternalFilterUpdateStatus=on  BusOutput=on
      settings: SourceProductBaseCode=VN
  CAN FD Receive2 : canfdlib/CAN FD Receive  BlockHandle=84680.0004  Device=Vector VN1640A 1 (Channel 4)  ObjConstructor=canChannel('Vector', 'VN1640A 1', 4, 'ProtocolMode', 'CAN FD')  EnableStandardIDsFilter=off  StdIDsCombo=Allow only  StandardIDs=1617  EnableExtendedIDsFilter=off  ExtIDsCombo=Allow all  ExtendedIDs=0  SampleTime=0.01  MsgsPerTimestep=all  InternalFilterUpdateStatus=on  BusOutput=on
      settings: SourceProductBaseCode=VN
  CAN FD Receive20 : canfdlib/CAN FD Receive  BlockHandle=84683.0004  Device=Vector VN1640A 1 (Channel 4)  ObjConstructor=canChannel('Vector', 'VN1640A 1', 4, 'ProtocolMode', 'CAN FD')  EnableStandardIDsFilter=off  StdIDsCombo=Allow only  StandardIDs=1635  EnableExtendedIDsFilter=off  ExtIDsCombo=Allow all  ExtendedIDs=0  SampleTime=0.01  MsgsPerTimestep=all  InternalFilterUpdateStatus=on  BusOutput=on
      settings: SourceProductBaseCode=VN
  CAN FD Receive21 : canfdlib/CAN FD Receive  BlockHandle=84686.0004  Device=Vector VN1640A 1 (Channel 4)  ObjConstructor=canChannel('Vector', 'VN1640A 1', 4, 'ProtocolMode', 'CAN FD')  EnableStandardIDsFilter=off  StdIDsCombo=Allow only  StandardIDs=1584  EnableExtendedIDsFilter=off  ExtIDsCombo=Allow all  ExtendedIDs=0  SampleTime=0.01  MsgsPerTimestep=all  InternalFilterUpdateStatus=on  BusOutput=on
      settings: SourceProductBaseCode=VN
  CAN FD Receive3 : canfdlib/CAN FD Receive  BlockHandle=84689.0004  Device=Vector VN1640A 1 (Channel 4)  ObjConstructor=canChannel('Vector', 'VN1640A 1', 4, 'ProtocolMode', 'CAN FD')  EnableStandardIDsFilter=off  StdIDsCombo=Allow only  StandardIDs=1618  EnableExtendedIDsFilter=off  ExtIDsCombo=Allow all  ExtendedIDs=0  SampleTime=0.01  MsgsPerTimestep=all  InternalFilterUpdateStatus=on  BusOutput=on
      settings: SourceProductBaseCode=VN
  CAN FD Receive4 : canfdlib/CAN FD Receive  BlockHandle=84692.0004  Device=Vector VN1640A 1 (Channel 4)  ObjConstructor=canChannel('Vector', 'VN1640A 1', 4, 'ProtocolMode', 'CAN FD')  EnableStandardIDsFilter=off  StdIDsCombo=Allow only  StandardIDs=1619  EnableExtendedIDsFilter=off  ExtIDsCombo=Allow all  ExtendedIDs=0  SampleTime=0.01  MsgsPerTimestep=all  InternalFilterUpdateStatus=on  BusOutput=on
      settings: SourceProductBaseCode=VN
  CAN FD Receive5 : canfdlib/CAN FD Receive  BlockHandle=84695.0004  Device=Vector VN1640A 1 (Channel 4)  ObjConstructor=canChannel('Vector', 'VN1640A 1', 4, 'ProtocolMode', 'CAN FD')  EnableStandardIDsFilter=off  StdIDsCombo=Allow only  StandardIDs=1620  EnableExtendedIDsFilter=off  ExtIDsCombo=Allow all  ExtendedIDs=0  SampleTime=0.01  MsgsPerTimestep=all  InternalFilterUpdateStatus=on  BusOutput=on
      settings: SourceProductBaseCode=VN
  CAN FD Receive6 : canfdlib/CAN FD Receive  BlockHandle=84698.0004  Device=Vector VN1640A 1 (Channel 4)  ObjConstructor=canChannel('Vector', 'VN1640A 1', 4, 'ProtocolMode', 'CAN FD')  EnableStandardIDsFilter=off  StdIDsCombo=Allow only  StandardIDs=1621  EnableExtendedIDsFilter=off  ExtIDsCombo=Allow all  ExtendedIDs=0  SampleTime=0.01  MsgsPerTimestep=all  InternalFilterUpdateStatus=on  BusOutput=on
      settings: SourceProductBaseCode=VN
  CAN FD Receive7 : canfdlib/CAN FD Receive  BlockHandle=84701.0004  Device=Vector VN1640A 1 (Channel 4)  ObjConstructor=canChannel('Vector', 'VN1640A 1', 4, 'ProtocolMode', 'CAN FD')  EnableStandardIDsFilter=off  StdIDsCombo=Allow only  StandardIDs=1622  EnableExtendedIDsFilter=off  ExtIDsCombo=Allow all  ExtendedIDs=0  SampleTime=0.01  MsgsPerTimestep=all  InternalFilterUpdateStatus=on  BusOutput=on
      settings: SourceProductBaseCode=VN
  CAN FD Receive8 : canfdlib/CAN FD Receive  BlockHandle=84704.0004  Device=Vector VN1640A 1 (Channel 4)  ObjConstructor=canChannel('Vector', 'VN1640A 1', 4, 'ProtocolMode', 'CAN FD')  EnableStandardIDsFilter=off  StdIDsCombo=Allow only  StandardIDs=1623  EnableExtendedIDsFilter=off  ExtIDsCombo=Allow all  ExtendedIDs=0  SampleTime=0.01  MsgsPerTimestep=all  InternalFilterUpdateStatus=on  BusOutput=on
      settings: SourceProductBaseCode=VN
  CAN FD Receive9 : canfdlib/CAN FD Receive  BlockHandle=84707.0004  Device=Vector VN1640A 1 (Channel 4)  ObjConstructor=canChannel('Vector', 'VN1640A 1', 4, 'ProtocolMode', 'CAN FD')  EnableStandardIDsFilter=off  StdIDsCombo=Allow only  StandardIDs=1624  EnableExtendedIDsFilter=off  ExtIDsCombo=Allow all  ExtendedIDs=0  SampleTime=0.01  MsgsPerTimestep=all  InternalFilterUpdateStatus=on  BusOutput=on
      settings: SourceProductBaseCode=VN
  Terminator{1..4,20,28,30..44} (21 alike) : Terminator
  VR_ADCU_IPM_ObjHeader_0x630FromInData : Outport
  VR_ADCU_IPM_Obj_01_0x650FromInData : Outport  Port=2
  VR_ADCU_IPM_Obj_02_0x651FromInData : Outport  Port=3
  VR_ADCU_IPM_Obj_03_0x652FromInData : Outport  Port=4
  VR_ADCU_IPM_Obj_04_0x653FromInData : Outport  Port=5
  VR_ADCU_IPM_Obj_05_0x654FromInData : Outport  Port=6
  VR_ADCU_IPM_Obj_06_0x655FromInData : Outport  Port=7
  VR_ADCU_IPM_Obj_07_0x656FromInData : Outport  Port=8
  VR_ADCU_IPM_Obj_08_0x657FromInData : Outport  Port=9
  VR_ADCU_IPM_Obj_09_0x658FromInData : Outport  Port=10
  VR_ADCU_IPM_Obj_10_0x659FromInData : Outport  Port=11
  VR_ADCU_IPM_Obj_11_0x65AFromInData : Outport  Port=12
  VR_ADCU_IPM_Obj_12_0x65BFromInData : Outport  Port=13
  VR_ADCU_IPM_Obj_13_0x65CFromInData : Outport  Port=14
  VR_ADCU_IPM_Obj_14_0x65DFromInData : Outport  Port=15
  VR_ADCU_IPM_Obj_15_0x65EFromInData : Outport  Port=16
  VR_ADCU_IPM_Obj_16_0x65FFromInData : Outport  Port=17
  VR_ADCU_IPM_Obj_17_0x660FromInData : Outport  Port=18
  VR_ADCU_IPM_Obj_18_0x661FromInData : Outport  Port=19
  VR_ADCU_IPM_Obj_19_0x662FromInData : Outport  Port=20
  VR_ADCU_IPM_Obj_20_0x663FromInData : Outport  Port=21
  wires:
  CAN FD Receive7/1 -> Terminator35/1
  CAN FD Receive11/2 -> VR_ADCU_IPM_Obj_11_0x65AFromInData/1
  CAN FD Receive10/1 -> Terminator38/1
  CAN FD Receive10/2 -> VR_ADCU_IPM_Obj_10_0x659FromInData/1
  CAN FD Receive9/1 -> Terminator37/1
  CAN FD Receive3/2 -> VR_ADCU_IPM_Obj_03_0x652FromInData/1
  CAN FD Receive2/2 -> VR_ADCU_IPM_Obj_02_0x651FromInData/1
  CAN FD Receive6/1 -> Terminator34/1
  CAN FD Receive16/2 -> VR_ADCU_IPM_Obj_16_0x65FFromInData/1
  CAN FD Receive15/1 -> Terminator43/1
  CAN FD Receive8/2 -> VR_ADCU_IPM_Obj_08_0x657FromInData/1
  CAN FD Receive1/1 -> Terminator28/1
  CAN FD Receive12/2 -> VR_ADCU_IPM_Obj_12_0x65BFromInData/1
  CAN FD Receive11/1 -> Terminator39/1
  CAN FD Receive7/2 -> VR_ADCU_IPM_Obj_07_0x656FromInData/1
  CAN FD Receive8/1 -> Terminator36/1
  CAN FD Receive14/2 -> VR_ADCU_IPM_Obj_14_0x65DFromInData/1
  CAN FD Receive13/1 -> Terminator41/1
  CAN FD Receive13/2 -> VR_ADCU_IPM_Obj_13_0x65CFromInData/1
  CAN FD Receive16/1 -> Terminator44/1
  CAN FD Receive1/2 -> VR_ADCU_IPM_Obj_01_0x650FromInData/1
  CAN FD Receive15/2 -> VR_ADCU_IPM_Obj_15_0x65EFromInData/1
  CAN FD Receive14/1 -> Terminator42/1
  CAN FD Receive9/2 -> VR_ADCU_IPM_Obj_09_0x658FromInData/1
  CAN FD Receive12/1 -> Terminator40/1
  CAN FD Receive6/2 -> VR_ADCU_IPM_Obj_06_0x655FromInData/1
  CAN FD Receive5/1 -> Terminator33/1
  CAN FD Receive4/2 -> VR_ADCU_IPM_Obj_04_0x653FromInData/1
  CAN FD Receive2/1 -> Terminator30/1
  CAN FD Receive3/1 -> Terminator31/1
  CAN FD Receive5/2 -> VR_ADCU_IPM_Obj_05_0x654FromInData/1
  CAN FD Receive4/1 -> Terminator32/1
  CAN FD Receive17/2 -> VR_ADCU_IPM_Obj_17_0x660FromInData/1
  CAN FD Receive17/1 -> Terminator1/1
  CAN FD Receive18/2 -> VR_ADCU_IPM_Obj_18_0x661FromInData/1
  CAN FD Receive18/1 -> Terminator2/1
  CAN FD Receive19/2 -> VR_ADCU_IPM_Obj_19_0x662FromInData/1
  CAN FD Receive19/1 -> Terminator3/1
  CAN FD Receive20/2 -> VR_ADCU_IPM_Obj_20_0x663FromInData/1
  CAN FD Receive20/1 -> Terminator4/1
  CAN FD Receive21/2 -> VR_ADCU_IPM_ObjHeader_0x630FromInData/1
  CAN FD Receive21/1 -> Terminator20/1

== system ALL_JP360_DBW_V6_5_1103/MsgFromCAN/MRR_Obj_data ==
  CAN FD Receive1 : canfdlib/CAN FD Receive  BlockHandle=84812.0006  Device=Vector VN1640A 1 (Channel 4)  ObjConstructor=canChannel('Vector', 'VN1640A 1', 4, 'ProtocolMode', 'CAN FD')  EnableStandardIDsFilter=off  StdIDsCombo=Allow only  StandardIDs=1680  EnableExtendedIDsFilter=off  ExtIDsCombo=Allow all  ExtendedIDs=0  SampleTime=0.01  MsgsPerTimestep=all  InternalFilterUpdateStatus=on  BusOutput=on
      settings: SourceProductBaseCode=VN
  CAN FD Receive10 : canfdlib/CAN FD Receive  BlockHandle=84815.0012  Device=Vector VN1640A 1 (Channel 4)  ObjConstructor=canChannel('Vector', 'VN1640A 1', 4, 'ProtocolMode', 'CAN FD')  EnableStandardIDsFilter=off  StdIDsCombo=Allow only  StandardIDs=1689  EnableExtendedIDsFilter=off  ExtIDsCombo=Allow all  ExtendedIDs=0  SampleTime=0.01  MsgsPerTimestep=all  InternalFilterUpdateStatus=on  BusOutput=on
      settings: SourceProductBaseCode=VN
  CAN FD Receive11 : canfdlib/CAN FD Receive  BlockHandle=84818.0006  Device=Vector VN1640A 1 (Channel 4)  ObjConstructor=canChannel('Vector', 'VN1640A 1', 4, 'ProtocolMode', 'CAN FD')  EnableStandardIDsFilter=off  StdIDsCombo=Allow only  StandardIDs=1690  EnableExtendedIDsFilter=off  ExtIDsCombo=Allow all  ExtendedIDs=0  SampleTime=0.01  MsgsPerTimestep=all  InternalFilterUpdateStatus=on  BusOutput=on
      settings: SourceProductBaseCode=VN
  CAN FD Receive12 : canfdlib/CAN FD Receive  BlockHandle=84821.0006  Device=Vector VN1640A 1 (Channel 4)  ObjConstructor=canChannel('Vector', 'VN1640A 1', 4, 'ProtocolMode', 'CAN FD')  EnableStandardIDsFilter=off  StdIDsCombo=Allow only  StandardIDs=1691  EnableExtendedIDsFilter=off  ExtIDsCombo=Allow all  ExtendedIDs=0  SampleTime=0.01  MsgsPerTimestep=all  InternalFilterUpdateStatus=on  BusOutput=on
      settings: SourceProductBaseCode=VN
  CAN FD Receive13 : canfdlib/CAN FD Receive  BlockHandle=84824.0005  Device=Vector VN1640A 1 (Channel 4)  ObjConstructor=canChannel('Vector', 'VN1640A 1', 4, 'ProtocolMode', 'CAN FD')  EnableStandardIDsFilter=off  StdIDsCombo=Allow only  StandardIDs=1692  EnableExtendedIDsFilter=off  ExtIDsCombo=Allow all  ExtendedIDs=0  SampleTime=0.01  MsgsPerTimestep=all  InternalFilterUpdateStatus=on  BusOutput=on
      settings: SourceProductBaseCode=VN
  CAN FD Receive14 : canfdlib/CAN FD Receive  BlockHandle=84827.0006  Device=Vector VN1640A 1 (Channel 4)  ObjConstructor=canChannel('Vector', 'VN1640A 1', 4, 'ProtocolMode', 'CAN FD')  EnableStandardIDsFilter=off  StdIDsCombo=Allow only  StandardIDs=1693  EnableExtendedIDsFilter=off  ExtIDsCombo=Allow all  ExtendedIDs=0  SampleTime=0.01  MsgsPerTimestep=all  InternalFilterUpdateStatus=on  BusOutput=on
      settings: SourceProductBaseCode=VN
  CAN FD Receive15 : canfdlib/CAN FD Receive  BlockHandle=84830.0006  Device=Vector VN1640A 1 (Channel 4)  ObjConstructor=canChannel('Vector', 'VN1640A 1', 4, 'ProtocolMode', 'CAN FD')  EnableStandardIDsFilter=off  StdIDsCombo=Allow only  StandardIDs=1694  EnableExtendedIDsFilter=off  ExtIDsCombo=Allow all  ExtendedIDs=0  SampleTime=0.01  MsgsPerTimestep=all  InternalFilterUpdateStatus=on  BusOutput=on
      settings: SourceProductBaseCode=VN
  CAN FD Receive16 : canfdlib/CAN FD Receive  BlockHandle=84833.0004  Device=Vector VN1640A 1 (Channel 4)  ObjConstructor=canChannel('Vector', 'VN1640A 1', 4, 'ProtocolMode', 'CAN FD')  EnableStandardIDsFilter=off  StdIDsCombo=Allow only  StandardIDs=1695  EnableExtendedIDsFilter=off  ExtIDsCombo=Allow all  ExtendedIDs=0  SampleTime=0.01  MsgsPerTimestep=all  InternalFilterUpdateStatus=on  BusOutput=on
      settings: SourceProductBaseCode=VN
  CAN FD Receive17 : canfdlib/CAN FD Receive  BlockHandle=84836.0004  Device=Vector VN1640A 1 (Channel 4)  ObjConstructor=canChannel('Vector', 'VN1640A 1', 4, 'ProtocolMode', 'CAN FD')  EnableStandardIDsFilter=off  StdIDsCombo=Allow only  StandardIDs=1664  EnableExtendedIDsFilter=off  ExtIDsCombo=Allow all  ExtendedIDs=0  SampleTime=0.01  MsgsPerTimestep=all  InternalFilterUpdateStatus=on  BusOutput=on
      settings: SourceProductBaseCode=VN
  CAN FD Receive2 : canfdlib/CAN FD Receive  BlockHandle=84839.0004  Device=Vector VN1640A 1 (Channel 4)  ObjConstructor=canChannel('Vector', 'VN1640A 1', 4, 'ProtocolMode', 'CAN FD')  EnableStandardIDsFilter=off  StdIDsCombo=Allow only  StandardIDs=1681  EnableExtendedIDsFilter=off  ExtIDsCombo=Allow all  ExtendedIDs=0  SampleTime=0.01  MsgsPerTimestep=all  InternalFilterUpdateStatus=on  BusOutput=on
      settings: SourceProductBaseCode=VN
  CAN FD Receive3 : canfdlib/CAN FD Receive  BlockHandle=84842.0004  Device=Vector VN1640A 1 (Channel 4)  ObjConstructor=canChannel('Vector', 'VN1640A 1', 4, 'ProtocolMode', 'CAN FD')  EnableStandardIDsFilter=off  StdIDsCombo=Allow only  StandardIDs=1682  EnableExtendedIDsFilter=off  ExtIDsCombo=Allow all  ExtendedIDs=0  SampleTime=0.01  MsgsPerTimestep=all  InternalFilterUpdateStatus=on  BusOutput=on
      settings: SourceProductBaseCode=VN
  CAN FD Receive4 : canfdlib/CAN FD Receive  BlockHandle=84845.0004  Device=Vector VN1640A 1 (Channel 4)  ObjConstructor=canChannel('Vector', 'VN1640A 1', 4, 'ProtocolMode', 'CAN FD')  EnableStandardIDsFilter=off  StdIDsCombo=Allow only  StandardIDs=1683  EnableExtendedIDsFilter=off  ExtIDsCombo=Allow all  ExtendedIDs=0  SampleTime=0.01  MsgsPerTimestep=all  InternalFilterUpdateStatus=on  BusOutput=on
      settings: SourceProductBaseCode=VN
  CAN FD Receive5 : canfdlib/CAN FD Receive  BlockHandle=84848.0004  Device=Vector VN1640A 1 (Channel 4)  ObjConstructor=canChannel('Vector', 'VN1640A 1', 4, 'ProtocolMode', 'CAN FD')  EnableStandardIDsFilter=off  StdIDsCombo=Allow only  StandardIDs=1684  EnableExtendedIDsFilter=off  ExtIDsCombo=Allow all  ExtendedIDs=0  SampleTime=0.01  MsgsPerTimestep=all  InternalFilterUpdateStatus=on  BusOutput=on
      settings: SourceProductBaseCode=VN
  CAN FD Receive6 : canfdlib/CAN FD Receive  BlockHandle=84851.0004  Device=Vector VN1640A 1 (Channel 4)  ObjConstructor=canChannel('Vector', 'VN1640A 1', 4, 'ProtocolMode', 'CAN FD')  EnableStandardIDsFilter=off  StdIDsCombo=Allow only  StandardIDs=1685  EnableExtendedIDsFilter=off  ExtIDsCombo=Allow all  ExtendedIDs=0  SampleTime=0.01  MsgsPerTimestep=all  InternalFilterUpdateStatus=on  BusOutput=on
      settings: SourceProductBaseCode=VN
  CAN FD Receive7 : canfdlib/CAN FD Receive  BlockHandle=84854.0004  Device=Vector VN1640A 1 (Channel 4)  ObjConstructor=canChannel('Vector', 'VN1640A 1', 4, 'ProtocolMode', 'CAN FD')  EnableStandardIDsFilter=off  StdIDsCombo=Allow only  StandardIDs=1686  EnableExtendedIDsFilter=off  ExtIDsCombo=Allow all  ExtendedIDs=0  SampleTime=0.01  MsgsPerTimestep=all  InternalFilterUpdateStatus=on  BusOutput=on
      settings: SourceProductBaseCode=VN
  CAN FD Receive8 : canfdlib/CAN FD Receive  BlockHandle=84857.0004  Device=Vector VN1640A 1 (Channel 4)  ObjConstructor=canChannel('Vector', 'VN1640A 1', 4, 'ProtocolMode', 'CAN FD')  EnableStandardIDsFilter=off  StdIDsCombo=Allow only  StandardIDs=1687  EnableExtendedIDsFilter=off  ExtIDsCombo=Allow all  ExtendedIDs=0  SampleTime=0.01  MsgsPerTimestep=all  InternalFilterUpdateStatus=on  BusOutput=on
      settings: SourceProductBaseCode=VN
  CAN FD Receive9 : canfdlib/CAN FD Receive  BlockHandle=84861.0004  Device=Vector VN1640A 1 (Channel 4)  ObjConstructor=canChannel('Vector', 'VN1640A 1', 4, 'ProtocolMode', 'CAN FD')  EnableStandardIDsFilter=off  StdIDsCombo=Allow only  StandardIDs=1688  EnableExtendedIDsFilter=off  ExtIDsCombo=Allow all  ExtendedIDs=0  SampleTime=0.01  MsgsPerTimestep=all  InternalFilterUpdateStatus=on  BusOutput=on
      settings: SourceProductBaseCode=VN
  Terminator{21,28,30..44} (17 alike) : Terminator
  VR_ADCU_MRR_ObjHeader_0x680FromInData : Outport
  VR_ADCU_MRR_Obj_01_02_0x690FromInData : Outport  Port=2
  VR_ADCU_MRR_Obj_03_04_0x691FromInData : Outport  Port=3
  VR_ADCU_MRR_Obj_05_06_0x692FromInData : Outport  Port=4
  VR_ADCU_MRR_Obj_07_08_0x693FromInData : Outport  Port=5
  VR_ADCU_MRR_Obj_09_10_0x694FromInData : Outport  Port=6
  VR_ADCU_MRR_Obj_11_12_0x695FromInData : Outport  Port=7
  VR_ADCU_MRR_Obj_13_14_0x696FromInData : Outport  Port=8
  VR_ADCU_MRR_Obj_15_16_0x697FromInData : Outport  Port=9
  VR_ADCU_MRR_Obj_17_18_0x698FromInData : Outport  Port=10
  VR_ADCU_MRR_Obj_19_20_0x699FromInData : Outport  Port=11
  VR_ADCU_MRR_Obj_21_22_0x69AFromInData : Outport  Port=12
  VR_ADCU_MRR_Obj_23_24_0x69BFromInData : Outport  Port=13
  VR_ADCU_MRR_Obj_25_26_0x69CFromInData : Outport  Port=14
  VR_ADCU_MRR_Obj_27_28_0x69DFromInData : Outport  Port=15
  VR_ADCU_MRR_Obj_29_30_0x69EFromInData : Outport  Port=16
  VR_ADCU_MRR_Obj_31_32_0x69FFromInData : Outport  Port=17
  wires:
  CAN FD Receive4/1 -> Terminator32/1
  CAN FD Receive5/2 -> VR_ADCU_MRR_Obj_09_10_0x694FromInData/1
  CAN FD Receive3/1 -> Terminator31/1
  CAN FD Receive2/1 -> Terminator30/1
  CAN FD Receive4/2 -> VR_ADCU_MRR_Obj_07_08_0x693FromInData/1
  CAN FD Receive5/1 -> Terminator33/1
  CAN FD Receive6/2 -> VR_ADCU_MRR_Obj_11_12_0x695FromInData/1
  CAN FD Receive12/1 -> Terminator40/1
  CAN FD Receive9/2 -> VR_ADCU_MRR_Obj_17_18_0x698FromInData/1
  CAN FD Receive14/1 -> Terminator42/1
  CAN FD Receive15/2 -> VR_ADCU_MRR_Obj_29_30_0x69EFromInData/1
  CAN FD Receive1/2 -> VR_ADCU_MRR_Obj_01_02_0x690FromInData/1
  CAN FD Receive16/1 -> Terminator44/1
  CAN FD Receive13/2 -> VR_ADCU_MRR_Obj_25_26_0x69CFromInData/1
  CAN FD Receive13/1 -> Terminator41/1
  CAN FD Receive14/2 -> VR_ADCU_MRR_Obj_27_28_0x69DFromInData/1
  CAN FD Receive8/1 -> Terminator36/1
  CAN FD Receive7/2 -> VR_ADCU_MRR_Obj_13_14_0x696FromInData/1
  CAN FD Receive11/1 -> Terminator39/1
  CAN FD Receive12/2 -> VR_ADCU_MRR_Obj_23_24_0x69BFromInData/1
  CAN FD Receive1/1 -> Terminator28/1
  CAN FD Receive8/2 -> VR_ADCU_MRR_Obj_15_16_0x697FromInData/1
  CAN FD Receive15/1 -> Terminator43/1
  CAN FD Receive16/2 -> VR_ADCU_MRR_Obj_31_32_0x69FFromInData/1
  CAN FD Receive6/1 -> Terminator34/1
  CAN FD Receive2/2 -> VR_ADCU_MRR_Obj_03_04_0x691FromInData/1
  CAN FD Receive3/2 -> VR_ADCU_MRR_Obj_05_06_0x692FromInData/1
  CAN FD Receive9/1 -> Terminator37/1
  CAN FD Receive10/2 -> VR_ADCU_MRR_Obj_19_20_0x699FromInData/1
  CAN FD Receive10/1 -> Terminator38/1
  CAN FD Receive11/2 -> VR_ADCU_MRR_Obj_21_22_0x69AFromInData/1
  CAN FD Receive7/1 -> Terminator35/1
  CAN FD Receive17/1 -> Terminator21/1
  CAN FD Receive17/2 -> VR_ADCU_MRR_ObjHeader_0x680FromInData/1
